simulink model "mg_test18"  (R2017b)
settings: Solver=VariableStepAuto  StartTime=0.0  StopTime=3  MaxStep=1e-4  RelTol=1e-3
values from neighbouring files (symbols this model uses):
  f = 50    [param_mgtest17.m]
  L = 0.15*Pbase/(2*pi*f)    (= 0.000459957785536)    [param_mgtest17.m]
  RL = 1.5e-3*Pbase    (= 0.001445)    [param_mgtest17.m]
  Ts_Power = 1/(fs*100)    (= 2.0202020202e-06)    [param_mgtest17.m]
libraries: powerlib x48, powerlib_meascontrol x15, simulink x8, re_lib x2, electricdrivelib x2, pePowerMeasurement x1
(part 2 of 2)

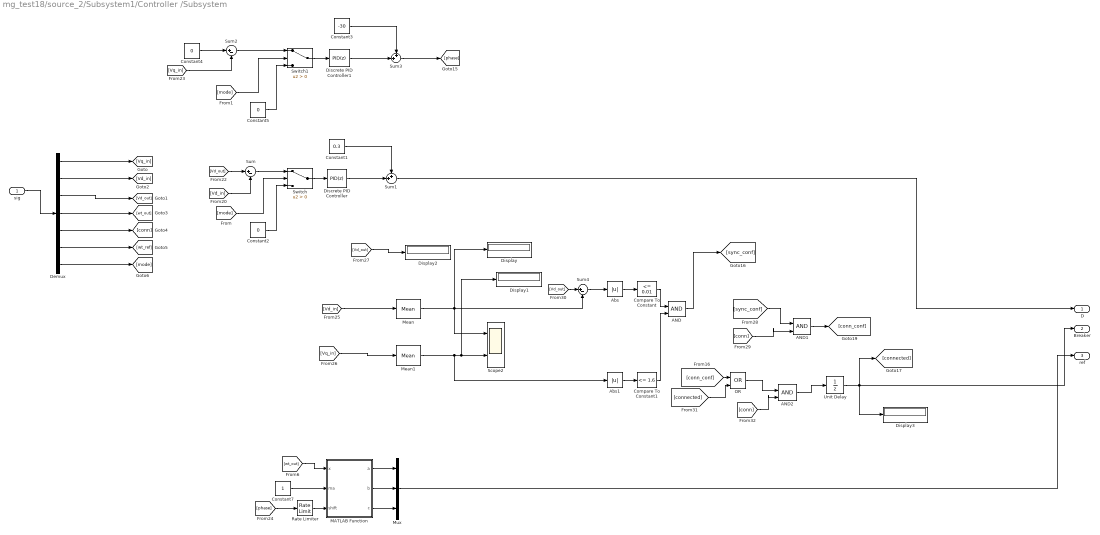
== system mg_test18/source_2/Subsystem1/Controller /Subsystem ==
  sig : Inport
  AND : Logic  IconShape=distinctive  AllPortsSameDT=off  OutDataTypeStr=boolean
  AND1 : Logic  IconShape=distinctive  AllPortsSameDT=off  OutDataTypeStr=boolean
  AND2 : Logic  IconShape=distinctive  AllPortsSameDT=off  OutDataTypeStr=boolean
  Abs : Abs
  Abs1 : Abs
  Compare To Constant : simulink/Logic and Bit Operations/Compare To Constant  relop=<=  const=0.01  OutDataTypeStr=boolean
  Compare To Constant1 : simulink/Logic and Bit Operations/Compare To Constant  relop=<=  const=1.6  OutDataTypeStr=boolean
  Constant1 : Constant  Value=0.3
  Constant2 : Constant  Value=0
  Constant3 : Constant  Value=-30
  Constant4 : Constant  Value=0
  Constant5 : Constant  Value=0
  Constant7 : Constant
  Demux : Demux  Outputs=7
  Discrete PID Controller : simulink/Continuous/PID Controller  Controller=PID  TimeDomain=Discrete-time  SampleTime=Ts_Power  IntegratorMethod=Forward Euler  FilterMethod=Forward Euler  Form=Parallel  UseFilter=on  ControllerParametersSource=internal  P=0.005  I=2  D=0  N=100  InitialConditionSource=internal  InitialConditionForIntegrator=0  InitialConditionForFilter=0  ExternalReset=none  LimitOutput=off  UpperSaturationLimit=inf  LowerSaturationLimit=-inf  LinearizeAsGain=off  AntiWindupMode=none  Kb=1  TrackingMode=off  Kt=1  PParamMin=[]  PParamMax=[]  IParamMin=[]  IParamMax=[]  DParamMin=[]  DParamMax=[]  NParamMin=[]  NParamMax=[]  KbParamMin=[]  KbParamMax=[]  KtParamMin=[]  KtParamMax=[]  POutMin=[]  POutMax=[]  IOutMin=[]  IOutMax=[]  DOutMin=[]  DOutMax=[]  NOutMin=[]  NOutMax=[]  KbOutMin=[]  KbOutMax=[]  KtOutMin=[]  KtOutMax=[]  IntegratorOutMin=[]  IntegratorOutMax=[]  FilterOutMin=[]  FilterOutMax=[]  SumOutMin=[]  SumOutMax=[]  SumI1OutMin=[]  SumI1OutMax=[]  SumI2OutMin=[]  SumI2OutMax=[]  SumI3OutMin=[]  SumI3OutMax=[]  SumDOutMin=[]  SumDOutMax=[]  SaturationOutMin=[]  SaturationOutMax=[]  IntegratorContinuousStateAttributes=''  IntegratorStateMustResolveToSignalObject=off  IntegratorRTWStateStorageClass=Auto  FilterContinuousStateAttributes=''  FilterStateMustResolveToSignalObject=off  FilterRTWStateStorageClass=Auto  DifferentiatorICPrevScaledInput=0  DifferentiatorOutMin=[]  DifferentiatorOutMax=[]  FilterDiffOutCoefMin=[]  FilterDiffOutCoefMax=[]  SumDenOutMin=[]  SumDenOutMax=[]  SumNumOutMin=[]  SumNumOutMax=[]  ReciprocalOutMin=[]  ReciprocalOutMax=[]  DivideOutMin=[]  DivideOutMax=[]  TunerSelectOption=Transfer Function Based (PID Tuner App)
  Discrete PID Controller1 : simulink/Continuous/PID Controller  Controller=PID  TimeDomain=Discrete-time  SampleTime=Ts_Power  IntegratorMethod=Forward Euler  FilterMethod=Forward Euler  Form=Parallel  UseFilter=on  ControllerParametersSource=internal  P=1  I=2  D=0  N=100  InitialConditionSource=internal  InitialConditionForIntegrator=0  InitialConditionForFilter=0  ExternalReset=none  LimitOutput=off  UpperSaturationLimit=inf  LowerSaturationLimit=-inf  LinearizeAsGain=off  AntiWindupMode=none  Kb=1  TrackingMode=off  Kt=1  PParamMin=[]  PParamMax=[]  IParamMin=[]  IParamMax=[]  DParamMin=[]  DParamMax=[]  NParamMin=[]  NParamMax=[]  KbParamMin=[]  KbParamMax=[]  KtParamMin=[]  KtParamMax=[]  POutMin=[]  POutMax=[]  IOutMin=[]  IOutMax=[]  DOutMin=[]  DOutMax=[]  NOutMin=[]  NOutMax=[]  KbOutMin=[]  KbOutMax=[]  KtOutMin=[]  KtOutMax=[]  IntegratorOutMin=[]  IntegratorOutMax=[]  FilterOutMin=[]  FilterOutMax=[]  SumOutMin=[]  SumOutMax=[]  SumI1OutMin=[]  SumI1OutMax=[]  SumI2OutMin=[]  SumI2OutMax=[]  SumI3OutMin=[]  SumI3OutMax=[]  SumDOutMin=[]  SumDOutMax=[]  SaturationOutMin=[]  SaturationOutMax=[]  IntegratorContinuousStateAttributes=''  IntegratorStateMustResolveToSignalObject=off  IntegratorRTWStateStorageClass=Auto  FilterContinuousStateAttributes=''  FilterStateMustResolveToSignalObject=off  FilterRTWStateStorageClass=Auto  DifferentiatorICPrevScaledInput=0  DifferentiatorOutMin=[]  DifferentiatorOutMax=[]  FilterDiffOutCoefMin=[]  FilterDiffOutCoefMax=[]  SumDenOutMin=[]  SumDenOutMax=[]  SumNumOutMin=[]  SumNumOutMax=[]  ReciprocalOutMin=[]  ReciprocalOutMax=[]  DivideOutMin=[]  DivideOutMax=[]  TunerSelectOption=Transfer Function Based (PID Tuner App)
  Display{,1..3} (4 alike) : Display
      Display settings: Decimation=4
      Display1 settings: Decimation=4
      Display2 settings: Decimation=4
  MATLAB Function : MATLAB Function  TreatAsAtomicUnit=on
  Mean : powerlib_meascontrol/Measurements/Mean  Freq=20  Vinit=0  Ts=0
  Mean1 : powerlib_meascontrol/Measurements/Mean  Freq=20  Vinit=5  Ts=0
  Mux : Mux  Inputs=3
  OR : Logic  Operator=OR  IconShape=distinctive  AllPortsSameDT=off  OutDataTypeStr=boolean
  Rate Limiter : RateLimiter  RisingSlewLimit=100  FallingSlewLimit=-100
  Scope2 : Scope  NumInputPorts=2
  Sum : Sum  Inputs=|+-
  Sum1 : Sum  Inputs=++|
  Sum2 : Sum  Inputs=|+-
  Sum3 : Sum  Inputs=++|
  Sum4 : Sum  Inputs=|+-
  Switch : Switch  Criteria=u2 > Threshold
  Switch1 : Switch  Criteria=u2 > Threshold
  Unit Delay : UnitDelay  SampleTime=Ts_Power
  D : Outport
  Breaker : Outport  Port=2
  ref : Outport  Port=3
  wires:
  Rate Limiter/1 -> MATLAB Function/3(shift)
  [Vd_in] -> Mean/1
  Sum1/1 -> D/1
  [Vq_in] -> Sum2/2
  MATLAB Function/3(c) -> Mux/3
  [Vd_out] -> Sum/1
  Mean/1 -> Sum4/2, Scope2/1, Display/1
  MATLAB Function/1(a) -> Mux/1
  Mean1/1 -> Abs1/1, Display1/1, Scope2/2
  Mux/1 -> ref/1
  [wt_out] -> MATLAB Function/1(x)
  Constant3/1 -> Sum3/1
  [connected] -> OR/2
  Sum4/1 -> Abs/1
  Constant4/1 -> Sum2/1
  AND2/1 -> Unit Delay/1
  AND/1 -> [sync_conf]
  Abs/1 -> Compare To Constant/1
  Constant7/1 -> MATLAB Function/2(ma)
  [Vd_in] -> Sum/2
  Sum3/1 -> [phase]
  Constant1/1 -> Sum1/1
  [Vd_out] -> Sum4/1
  [sync_conf] -> AND1/1
  MATLAB Function/2(b) -> Mux/2
  Abs1/1 -> Compare To Constant1/1
  Compare To Constant1/1 -> AND/2
  [Vq_in] -> Mean1/1
  Discrete PID Controller1/1 -> Sum3/2
  [Vd_out] -> Display2/1
  Compare To Constant/1 -> AND/1
  Unit Delay/1 -> Breaker/1, Display3/1, [connected]
  Discrete PID Controller/1 -> Sum1/2
  AND1/1 -> [conn_conf]
  [conn] -> AND1/2
  [conn] -> AND2/2
  [phase] -> Rate Limiter/1
  OR/1 -> AND2/1
  [conn_conf] -> OR/1
  Demux/1 -> [Vq_in]
  Demux/3 -> [Vd_out]
  Demux/2 -> [Vd_in]
  Demux/4 -> [wt_out]
  sig/1 -> Demux/1
  Demux/5 -> [conn]
  Demux/6 -> [wt_ref]
  Demux/7 -> [mode]
  Sum/1 -> Switch/1
  Switch/1 -> Discrete PID Controller/1
  Constant2/1 -> Switch/3
  [mode] -> Switch/2
  [mode] -> Switch1/2
  Constant5/1 -> Switch1/3
  Switch1/1 -> Discrete PID Controller1/1
  Sum2/1 -> Switch1/1

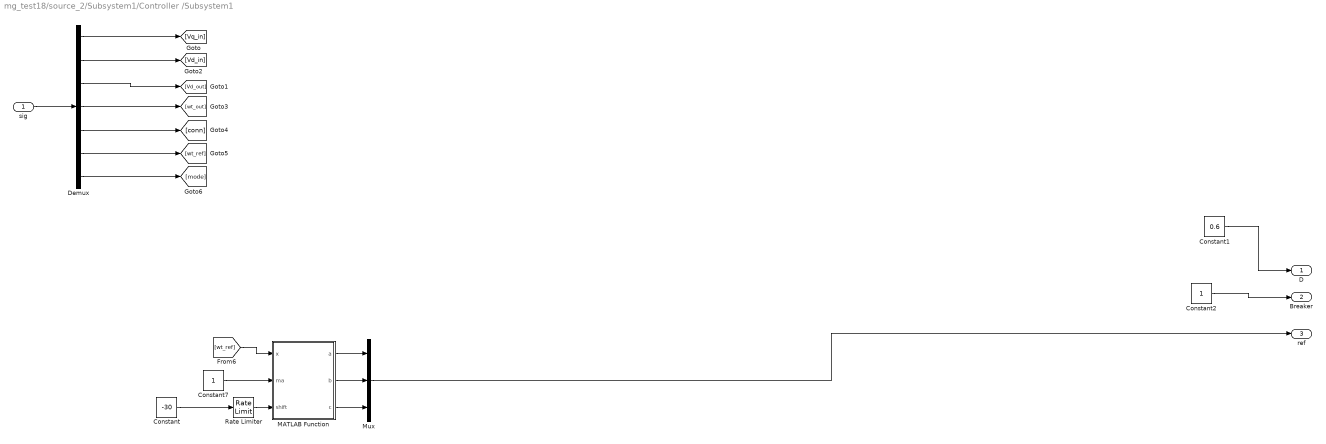
== system mg_test18/source_2/Subsystem1/Controller /Subsystem1 ==
  sig : Inport
  Constant : Constant  Value=-30
  Constant1 : Constant  Value=0.6
  Constant2 : Constant
  Constant7 : Constant
  Demux : Demux  Outputs=7
  MATLAB Function : MATLAB Function  TreatAsAtomicUnit=on
  Mux : Mux  Inputs=3
  Rate Limiter : RateLimiter  RisingSlewLimit=100  FallingSlewLimit=-100
  D : Outport
  Breaker : Outport  Port=2
  ref : Outport  Port=3
  wires:
  Rate Limiter/1 -> MATLAB Function/3(shift)
  MATLAB Function/3(c) -> Mux/3
  MATLAB Function/1(a) -> Mux/1
  Mux/1 -> ref/1
  [wt_ref] -> MATLAB Function/1(x)
  Constant7/1 -> MATLAB Function/2(ma)
  MATLAB Function/2(b) -> Mux/2
  Constant/1 -> Rate Limiter/1
  Constant1/1 -> D/1
  Demux/5 -> [conn]
  sig/1 -> Demux/1
  Demux/2 -> [Vd_in]
  Demux/1 -> [Vq_in]
  Demux/7 -> [mode]
  Demux/4 -> [wt_out]
  Demux/6 -> [wt_ref]
  Demux/3 -> [Vd_out]
  Constant2/1 -> Breaker/1

== matlab function mg_test18/source_1/Subsystem1/Controller /Subsystem1/MATLAB Function ==
  data: x input; a output; ma input; shift input; b output; c output
function [a,b,c] = ref_generation(x,ma,shift)

shift_k = shift*pi/180;
a = (ma*sin((x) + shift_k));
b = (ma*sin((x)+shift_k-(2*pi/3)));
c = (ma*sin((x)+shift_k+(2*pi/3)));

== matlab function mg_test18/source_1/Subsystem1/Controller /Subsystem/MATLAB Function ==
  data: x input; a output; ma input; shift input; b output; c output
function [a,b,c] = ref_generation(x,ma,shift)

shift_k = shift*pi/180;
a = (ma*sin((x) + shift_k));
b = (ma*sin((x)+shift_k-(2*pi/3)));
c = (ma*sin((x)+shift_k+(2*pi/3)));

== matlab function mg_test18/source_2/Subsystem1/Controller /Subsystem/MATLAB Function ==
  data: x input; a output; ma input; shift input; b output; c output
function [a,b,c] = ref_generation(x,ma,shift)

shift_k = shift*pi/180;
a = (ma*sin((x) + shift_k));
b = (ma*sin((x)+shift_k-(2*pi/3)));
c = (ma*sin((x)+shift_k+(2*pi/3)));

== matlab function mg_test18/source_2/Subsystem1/Controller /Subsystem1/MATLAB Function ==
  data: x input; a output; ma input; shift input; b output; c output
function [a,b,c] = ref_generation(x,ma,shift)

shift_k = shift*pi/180;
a = (ma*sin((x) + shift_k));
b = (ma*sin((x)+shift_k-(2*pi/3)));
c = (ma*sin((x)+shift_k+(2*pi/3)));
